simulink model "SIM_NonlinearPIwAW_2017b"  (R2017b)
settings: Solver=FixedStepAuto  StartTime=0.0  StopTime=9*0.25  FixedStep=h  RelTol=1e-3
values from neighbouring files (symbols this model uses):
  h = 1e-5    (= 1e-05)    [init.m]
  J = [0 -1; 1 0]    [generate_EKF.m]    (also in init.m)
  log_ts = 1e-5    (= 1e-05)    [init.m]
  lut_fr =     [friction.mat]
  omegam_ref = 157    [init.m]
  p = 2    [generate_EKF.m]
  P_init_dist = W_dist_noise    [init.m]
  pmsm_sew =     [config.mat]
  Psi_jac = [0.121, 0; 0, 0.0769]    [init.m]
  rsm_za =     [config.mat]
  SysConfig_SamplingTimeA = 0.00025    [config.mat]
  SysConfig_SamplingTimeB = 0.00025    [config.mat]
  u_DC = 556    [init.m]
  V_dist_noise = diag([2e0, 2e0])    [init.m]
  W_dist_noise = diag([1e-2, 1e-2, 1e4, 1e4])    [init.m]
  x_e_init_dist = zeros(4,1)    [init.m]
undefined symbols (not defined in the file or in its folder): DiscIntNeverNeededParam, f_pwm, k_i, k_p_tilde, uhat
libraries: simulink x4
(part 1 of 2)
settings Model: Creator=Julian Kullick  LastModifiedBy=andrea
settings DataIOCC: SaveFormat=StructureWithTime  SaveOutput=off  DSMLogging=off  SaveTime=off  SignalLoggingName=simData  LoggingFileName=./results/sim/NonlinearPIwAW.mat
settings SFSimCC: SimUseLocalCustomCode=on
settings RTWCC: RTWUseLocalCustomCode=on

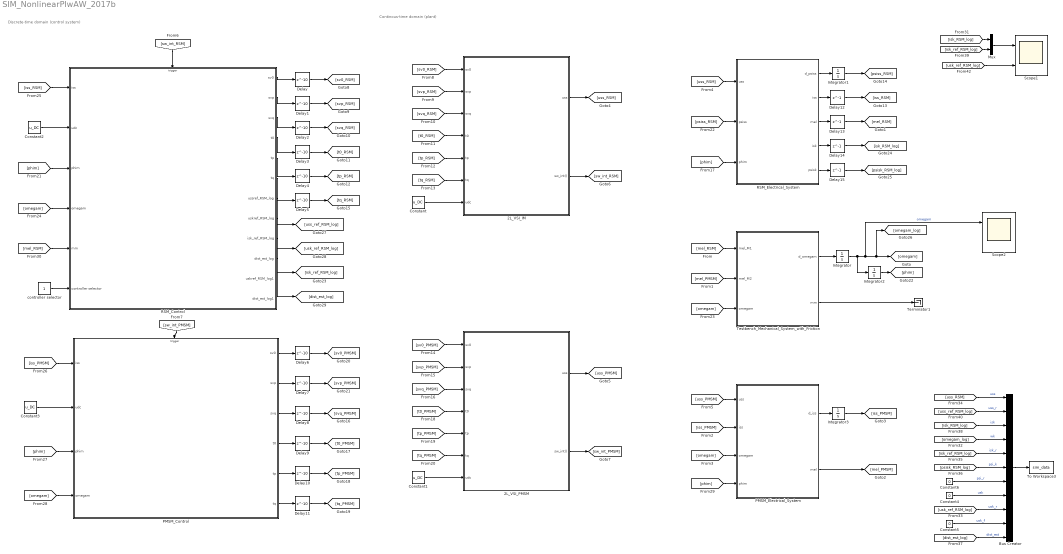
== system SIM_NonlinearPIwAW_2017b ==
  note: Continous-time domain (plant)
  note: Discrete-time domain (control system)
  2L_VSI_IM : Subsystem  mask{TS=SysConfig_SamplingTimeA, H=h}
      mask prompts: TS "PWM period (symmetric sampling)"; H "Model sampling time"
      mask DialogControl DescGroupVar Prompt: Description
      mask DialogControl DescTextVar Prompt: 2-level VSI output generator.
  2L_VSI_PMSM : Subsystem  mask{TS=SysConfig_SamplingTimeB, H=h}
      mask prompts: TS "PWM period (symmetric sampling)"; H "Model sampling time"
      mask DialogControl DescGroupVar Prompt: Description
      mask DialogControl DescTextVar Prompt: 2-level VSI output generator.
  Bus Creator : BusCreator  Inputs=11
  Constant{,1..3} (4 alike) : Constant  Value=u_DC
  Constant4 : Constant  Value=0
  Constant5 : Constant  Value=0
  Constant6 : Constant  Value=0
  Delay{,1..11} (12 alike) : Delay  DelayLength=10
  Delay{12..15} (4 alike) : Delay  DelayLength=1
  Integrator{,1..3} (4 alike) : Integrator
  Mux : Mux  Inputs=2
  PMSM_Control : Subsystem  TreatAsAtomicUnit=on
  PMSM_Electrical_System : MATLAB Function  TreatAsAtomicUnit=on  mask{RS=pmsm_sew.Rs, LS=pmsm_sew.Ls, PSIPM=pmsm_sew.PsiPM, NP=pmsm_sew.np}
      mask prompts: RS "Stator resistance (in Ohm)"; LS "Stator inductance (in H)"; PSIPM "Permanent magnet flux (in Wb)"; NP "Number of pole pairs"
  RSM_Control : Subsystem  TreatAsAtomicUnit=on
  RSM_Electrical_System : MATLAB Function  TreatAsAtomicUnit=on  mask{RS=rsm_za.Rs, NP=rsm_za.np, ISD=rsm_za.Is.d, ISQ=rsm_za.Is.q, PSISD=rsm_za.Psis.d, PSISQ=rsm_za.Psis.q}
      mask prompts: RS "Stator resistance (in Ohm)"; NP "Number of pole pairs"; ISD "d-Current for flux look-up (in A) [VEC]"; ISQ "q-Current for flux look-up (in A) [VEC]"; PSISD "d-Flux map (in Wb) [MAP]"; PSISQ "q-Flux map (in Wb) [MAP]|"
  Scope1 : Scope  NumInputPorts=2
  Scope2 : Scope  NumInputPorts=2
  Terminator1 : Terminator
  Testbench_Mechanical_System_with_Friction : MATLAB Function  TreatAsAtomicUnit=on  mask{THETAM_M1=rsm_za.Thetam, THETAM_M2=pmsm_sew.Thetam, MFR_LUT=lut_fr.m*0, WFR_LUT=lut_fr.omega}
      mask prompts: THETAM_M1 "Moment of inertia of machine 1 (in kg m^2)"; THETAM_M2 "Moment of inertia of machine 2 (in kg m^2)"; MFR_LUT "Friction torque [VEC] (in Nm)"; WFR_LUT "Speed vector for torque look-up [VEC] (in rad/s)"
  To Workspace3 : ToWorkspace  VariableName=sim_data  SaveFormat=Timeseries  SampleTime=log_ts
  controller selector : Constant
  wires:
  RSM_Electrical_System/1(d_psiss) -> Integrator1/1
  [phim] -> RSM_Electrical_System/3(phim)
  Integrator1/1 -> [psiss_RSM]
  RSM_Electrical_System/3(mel) -> Delay13/1
  [psiss_RSM] -> RSM_Electrical_System/2(psiss)
  Testbench_Mechanical_System_with_Friction/1(d_omegam) -> Integrator/1
  Integrator2/1 -> [phim]
  Testbench_Mechanical_System_with_Friction/2(mm) -> Terminator1/1
  PMSM_Electrical_System/2(mel) -> [mel_PMSM]
  Integrator3/1 -> [iss_PMSM]
  PMSM_Electrical_System/1(d_iss) -> Integrator3/1
  [iss_PMSM] -> PMSM_Electrical_System/2(iss)
  [omegam] -> PMSM_Electrical_System/3(omegam)
  2L_VSI_IM/1(uss) -> [uss_RSM]
  [uss_RSM] -> RSM_Electrical_System/1(uss)
  2L_VSI_PMSM/1(uss) -> [uss_PMSM]
  [uss_PMSM] -> PMSM_Electrical_System/1(uss)
  2L_VSI_IM/2(sw_int()) -> [sw_int_RSM]
  [sw_int_PMSM] -> PMSM_Control/Trigger
  2L_VSI_PMSM/2(sw_int()) -> [sw_int_PMSM]
  [sw_int_RSM] -> RSM_Control/Trigger
  RSM_Control/1(sv0) -> Delay/1
  RSM_Control/2(svp) -> Delay1/1
  RSM_Control/3(svq) -> Delay2/1
  RSM_Control/4(t0) -> Delay3/1
  RSM_Control/5(tp) -> Delay4/1
  RSM_Control/6(tq) -> Delay5/1
  [t0_RSM] -> 2L_VSI_IM/4(t0)
  [tq_RSM] -> 2L_VSI_IM/6(tq)
  [tp_RSM] -> 2L_VSI_IM/5(tp)
  [svq_RSM] -> 2L_VSI_IM/3(svq)
  [svp_RSM] -> 2L_VSI_IM/2(svp)
  [sv0_RSM] -> 2L_VSI_IM/1(sv0)
  Constant/1 -> 2L_VSI_IM/7(udc)
  PMSM_Control/1(sv0) -> Delay6/1
  PMSM_Control/2(svp) -> Delay7/1
  PMSM_Control/3(svq) -> Delay8/1
  PMSM_Control/4(t0) -> Delay9/1
  PMSM_Control/5(tp) -> Delay10/1
  PMSM_Control/6(tq) -> Delay11/1
  [sv0_PMSM] -> 2L_VSI_PMSM/1(sv0)
  [svp_PMSM] -> 2L_VSI_PMSM/2(svp)
  [svq_PMSM] -> 2L_VSI_PMSM/3(svq)
  [t0_PMSM] -> 2L_VSI_PMSM/4(t0)
  [tp_PMSM] -> 2L_VSI_PMSM/5(tp)
  [tq_PMSM] -> 2L_VSI_PMSM/6(tq)
  Constant1/1 -> 2L_VSI_PMSM/7(udc)
  [omegam] -> Testbench_Mechanical_System_with_Friction/3(omegam)
  Constant2/1 -> RSM_Control/2(udc)
  [omegam] -> RSM_Control/4(omegam)
  [iss_RSM] -> RSM_Control/1(iss)
  [iss_PMSM] -> PMSM_Control/1(iss)
  Constant3/1 -> PMSM_Control/2(udc)
  [phim] -> PMSM_Control/3(phim)
  [omegam] -> PMSM_Control/4(omegam)
  Integrator/1 -> Integrator2/1, Scope2/1, [omegam_log], [omegam]  "omegam"
  [mel_RSM] -> Testbench_Mechanical_System_with_Friction/1(mel_M1)
  [mel_PMSM] -> Testbench_Mechanical_System_with_Friction/2(mel_M2)
  [phim] -> PMSM_Electrical_System/4(phim)
  RSM_Electrical_System/2(iss) -> Delay12/1
  Delay/1 -> [sv0_RSM]
  Delay1/1 -> [svp_RSM]
  Delay2/1 -> [svq_RSM]
  Delay3/1 -> [t0_RSM]
  Delay4/1 -> [tp_RSM]
  Delay5/1 -> [tq_RSM]
  Delay6/1 -> [sv0_PMSM]
  Delay7/1 -> [svp_PMSM]
  Delay8/1 -> [svq_PMSM]
  Delay9/1 -> [t0_PMSM]
  Delay10/1 -> [tp_PMSM]
  Delay11/1 -> [tq_PMSM]
  Delay12/1 -> [iss_RSM]
  [phim] -> RSM_Control/3(phim)
  [mel_RSM] -> RSM_Control/5(mm)
  Delay13/1 -> [mel_RSM]
  controller selector/1 -> RSM_Control/6(controller selector)
  RSM_Electrical_System/4(isk) -> Delay14/1
  Delay14/1 -> [isk_RSM_log]
  RSM_Electrical_System/5(psisk) -> Delay15/1
  Delay15/1 -> [psisk_RSM_log]
  RSM_Control/7(ussref_RSM_log) -> [uss_ref_RSM_log]
  RSM_Control/8(uskref_RSM_log) -> [usk_ref_RSM_log]
  RSM_Control/9(isk_ref_RSM_log) -> [isk_ref_RSM_log]
  RSM_Control/10(dist_est_log) -> [dist_est_log]
  [isk_RSM_log] -> Mux/1
  [isk_ref_RSM_log] -> Mux/2
  [usk_ref_RSM_log] -> Scope1/2
  Mux/1 -> Scope1/1
  Bus Creator/1 -> To Workspace3/1
  [uss_RSM] -> Bus Creator/1  "uss"
  [uss_ref_RSM_log] -> Bus Creator/2  "uss_r"
  [isk_RSM_log] -> Bus Creator/3  "isk"
  [omegam_log] -> Bus Creator/4  "wk"
  [isk_ref_RSM_log] -> Bus Creator/5  "isk_r"
  [psisk_RSM_log] -> Bus Creator/6  "psi_k"
  Constant6/1 -> Bus Creator/7  "psi_r"
  Constant4/1 -> Bus Creator/8  "usk"
  [usk_ref_RSM_log] -> Bus Creator/9  "usk_r"
  Constant5/1 -> Bus Creator/10  "usk_f"
  [dist_est_log] -> Bus Creator/11  "dist_est"

== system SIM_NonlinearPIwAW_2017b/2L_VSI_IM ==
  sv0 : Inport
  svp : Inport  Port=2
  svq : Inport  Port=3
  t0 : Inport  Port=4
  tp : Inport  Port=5
  tq : Inport  Port=6
  udc : Inport  Port=7
  NL_VSI : Subsystem  mask{N=2, TPWM=TS, HSIM=H, INT_SHIFT=0}
      mask prompts: N "Number of levels"; TPWM "PWM period (symmetrical PWM)"; HSIM "Model sampling time"; INT_SHIFT "Interrupt shift (in percent of cycle time)"
      mask init:
      | INT_OFFSET = floor(TPWM/HSIM*INT_SHIFT*0.01);
      mask DialogControl DescTextVar Prompt: N-level VSI output signal generator.
  TC : Gain  Gain=2/3*[1 -0.5 -0.5; 0 sqrt(3)/2 -sqrt(3)/2]  Multiplication=Matrix(K*u)
  Terminator : Terminator
  uss : Outport
  sw_int() : Outport  Port=2
  wires:
  NL_VSI/3(sw_int()) -> sw_int()/1
  udc/1 -> NL_VSI/7(udc)
  NL_VSI/1(uabc0) -> TC/1
  sv0/1 -> NL_VSI/1(sv0)
  svp/1 -> NL_VSI/2(svp)
  svq/1 -> NL_VSI/3(svq)
  t0/1 -> NL_VSI/4(t0)
  tp/1 -> NL_VSI/5(tp)
  tq/1 -> NL_VSI/6(tq)
  TC/1 -> uss/1
  NL_VSI/2(ucm) -> Terminator/1

== system SIM_NonlinearPIwAW_2017b/2L_VSI_PMSM ==
  sv0 : Inport
  svp : Inport  Port=2
  svq : Inport  Port=3
  t0 : Inport  Port=4
  tp : Inport  Port=5
  tq : Inport  Port=6
  udc : Inport  Port=7
  NL_VSI : Subsystem  mask{N=2, TPWM=TS, HSIM=H, INT_SHIFT=0}
      mask prompts: N "Number of levels"; TPWM "PWM period (symmetrical PWM)"; HSIM "Model sampling time"; INT_SHIFT "Interrupt shift (in percent of cycle time)"
      mask init:
      | INT_OFFSET = floor(TPWM/HSIM*INT_SHIFT*0.01);
      mask DialogControl DescTextVar Prompt: N-level VSI output signal generator.
  TC : Gain  Gain=2/3*[1 -0.5 -0.5; 0 sqrt(3)/2 -sqrt(3)/2]  Multiplication=Matrix(K*u)
  Terminator : Terminator
  uss : Outport
  sw_int() : Outport  Port=2
  wires:
  NL_VSI/3(sw_int()) -> sw_int()/1
  udc/1 -> NL_VSI/7(udc)
  NL_VSI/1(uabc0) -> TC/1
  sv0/1 -> NL_VSI/1(sv0)
  svp/1 -> NL_VSI/2(svp)
  svq/1 -> NL_VSI/3(svq)
  t0/1 -> NL_VSI/4(t0)
  tp/1 -> NL_VSI/5(tp)
  tq/1 -> NL_VSI/6(tq)
  TC/1 -> uss/1
  NL_VSI/2(ucm) -> Terminator/1

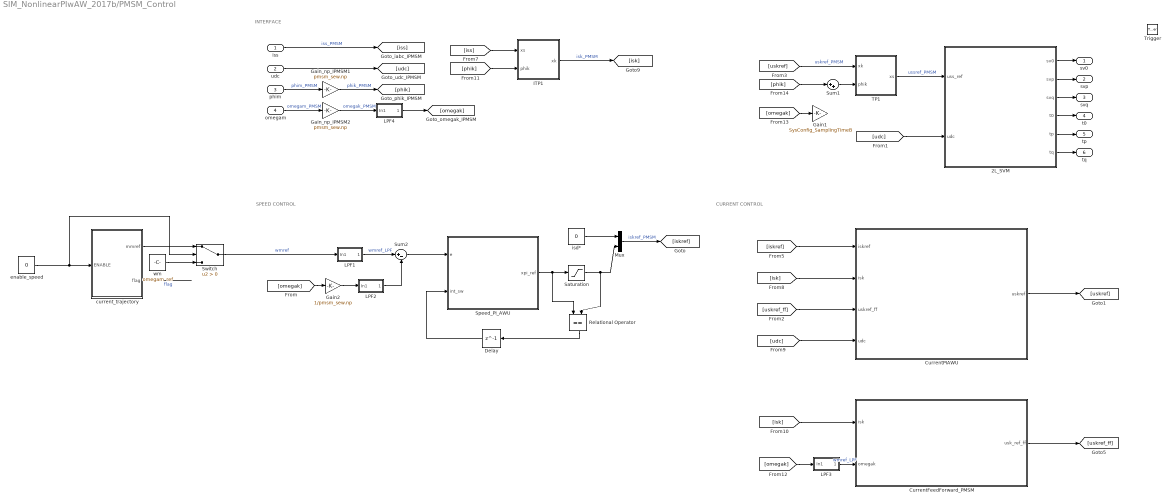
== system SIM_NonlinearPIwAW_2017b/PMSM_Control ==
  note: CURRENT CONTROL
  note: SPEED CONTROL
  note: INTERFACE
  iss : Inport
  udc : Inport  Port=2
  phim : Inport  Port=3
  omegam : Inport  Port=4
  Trigger : TriggerPort  TriggerType=function-call  VariantControl=Variant
  2L_SVM : Subsystem  mask{TS=SysConfig_SamplingTimeA}
      mask prompts: TS "PWM period (symmetric sampling)"
      mask DialogControl DescGroupVar Prompt: Description
      mask DialogControl DescTextVar Prompt: 2-level space vector modulator.
  CurrentFeedForward_PMSM : MATLAB Function  TreatAsAtomicUnit=on
  CurrentPIAWU : Subsystem  mask{VRD=pmsm_sew.VRis, TND=pmsm_sew.Tnis, VRQ=pmsm_sew.VRis, TNQ=pmsm_sew.Tnis}
      mask prompts: VRD "d-Current gain (constant part)"; TND "d-Current time constant (constant part)"; VRQ "q-Current gain (constant part)"; TNQ "q-Current time constant (constant part)"
      mask DialogControl DescGroupVar Prompt: Description
      mask DialogControl DescTextVar Prompt: Current control system with anti windup and online parameter adjustment.
  Delay : Delay  DelayLength=1
  Gain1 : Gain  Gain=SysConfig_SamplingTimeB
  Gain2 : Gain  Gain=1/pmsm_sew.np
  Gain_np_IPMSM1 : Gain  Gain=pmsm_sew.np
  Gain_np_IPMSM2 : Gain  Gain=pmsm_sew.np
  ITP1 : MATLAB Function  TreatAsAtomicUnit=on
  LPF1 : Subsystem  mask{TF=SysConfig_SamplingTimeB*100, TS=SysConfig_SamplingTimeB, SAT=inf}
      mask prompts: TF "Filter constant"; TS "Sampling time"; SAT "Saturation"
  LPF2 : Subsystem  mask{TF=SysConfig_SamplingTimeB*20, TS=SysConfig_SamplingTimeB, SAT=inf}
      mask prompts: TF "Filter constant"; TS "Sampling time"; SAT "Saturation"
  LPF3 : Subsystem  mask{TF=SysConfig_SamplingTimeB*10, TS=SysConfig_SamplingTimeB, SAT=350}
      mask prompts: TF "Filter constant"; TS "Sampling time"; SAT "Saturation"
  LPF4 : Subsystem  mask{TF=SysConfig_SamplingTimeB*32, TS=SysConfig_SamplingTimeB, SAT=inf}
      mask prompts: TF "Filter constant"; TS "Sampling time"; SAT "Saturation"
  Mux : Mux  Inputs=2
  Relational Operator : RelationalOperator  Operator===  OutDataTypeStr=boolean  RndMeth=Simplest
  Saturation : Saturate  UpperLimit=pmsm_sew.ishatN*1.2  LowerLimit=-pmsm_sew.ishatN*1.2
  Speed_PI_AWU : Subsystem  mask{VR=pmsm_sew.VRomegam*0.25, TN=pmsm_sew.Tnomegam*25}
      mask prompts: VR "Gain"; TN "Time constant (in s)"
  Sum1 : Sum  Inputs=|++
  Sum2 : Sum  Inputs=|+-
  Switch : Switch  Criteria=u2 > Threshold
  TP1 : MATLAB Function  TreatAsAtomicUnit=on
  current_trajectory : Subsystem
  enable_speed : Constant  Value=0
  isd* : Constant  Value=0
  wm : Constant  Value=omegam_ref
  sv0 : Outport
  svp : Outport  Port=2
  svq : Outport  Port=3
  t0 : Outport  Port=4
  tp : Outport  Port=5
  tq : Outport  Port=6
  wires:
  [omegak] -> LPF3/1(In1)
  Delay/1 -> Speed_PI_AWU/2(int_sw)
  [isk] -> CurrentPIAWU/2(isk)
  CurrentPIAWU/1(uskref) -> [uskref]
  Switch/1 -> LPF1/1(In1)  "wmref"
  [udc] -> CurrentPIAWU/4(udc)
  Speed_PI_AWU/1(xpi_ref) -> Relational Operator/1, Saturation/1
  [isk] -> CurrentFeedForward_PMSM/1(isk)
  Sum2/1 -> Speed_PI_AWU/1(e)
  Saturation/1 -> Relational Operator/2, Mux/2
  [uskref_ff] -> CurrentPIAWU/3(uskref_ff)
  [omegak] -> Gain2/1
  isd*/1 -> Mux/1
  CurrentFeedForward_PMSM/1(usk_ref_ff) -> [uskref_ff]
  Relational Operator/1 -> Delay/1
  2L_SVM/6(tq) -> tq/1
  2L_SVM/2(svp) -> svp/1
  2L_SVM/3(svq) -> svq/1
  2L_SVM/4(t0) -> t0/1
  2L_SVM/1(sv0) -> sv0/1
  2L_SVM/5(tp) -> tp/1
  Sum1/1 -> TP1/2(phik)
  ITP1/1(xk) -> [isk]  "isk_PMSM"
  [uskref] -> TP1/1(xk)  "uskref_PMSM"
  [phik] -> Sum1/1
  [phik] -> ITP1/2(phik)
  Gain_np_IPMSM1/1 -> [phik]  "phik_PMSM"
  [omegak] -> Gain1/1
  Gain_np_IPMSM2/1 -> LPF4/1(In1)  "omegak_PMSM"
  iss/1 -> [iss]  "iss_PMSM"
  [iss] -> ITP1/1(xs)
  udc/1 -> [udc]
  phim/1 -> Gain_np_IPMSM1/1  "phim_PMSM"
  omegam/1 -> Gain_np_IPMSM2/1  "omegam_PMSM"
  [udc] -> 2L_SVM/2(udc)
  TP1/1(xs) -> 2L_SVM/1(uss_ref)  "ussref_PMSM"
  Mux/1 -> [iskref]  "iskref_PMSM"
  Gain2/1 -> LPF2/1(In1)
  [iskref] -> CurrentPIAWU/1(iskref)
  LPF1/1(Out1) -> Sum2/1  "wmref_LPF"
  LPF2/1(Out1) -> Sum2/2
  current_trajectory/2(flag) -> ?  "flag"
  wm/1 -> Switch/3
  current_trajectory/1(mmref) -> Switch/1
  enable_speed/1 -> Switch/2, current_trajectory/1(ENABLE)
  LPF3/1(Out1) -> CurrentFeedForward_PMSM/2(omegak)  "wmref_LPF"
  LPF4/1(Out1) -> [omegak]

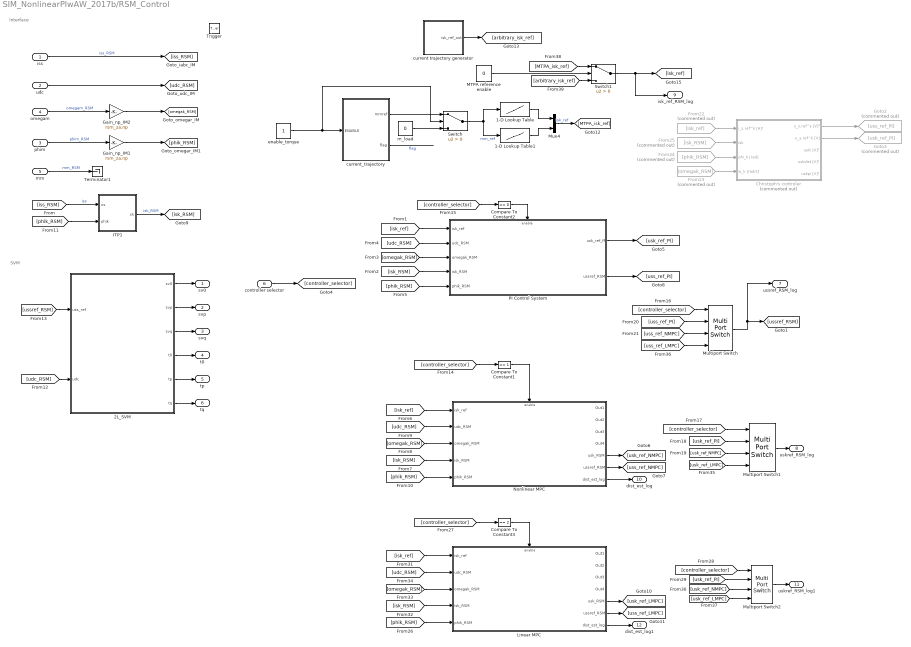
== system SIM_NonlinearPIwAW_2017b/RSM_Control ==
  note: SVM
  note: Interface
  iss : Inport
  udc : Inport  Port=2
  phim : Inport  Port=3
  omegam : Inport  Port=4
  mm : Inport  Port=5
  controller selector : Inport  Port=6
  Trigger : TriggerPort  TriggerType=function-call  VariantControl=Variant
  1-D Lookup Table : Lookup_n-D  NumberOfTableDimensions=1  BreakpointsForDimension1=rsm_za.MTPA.mm  Table=rsm_za.MTPA.d  RemoveProtectionInput=on  InternalRulePriority=Speed  RndMeth=Simplest  InputSameDT=on
  1-D Lookup Table1 : Lookup_n-D  NumberOfTableDimensions=1  BreakpointsForDimension1=rsm_za.MTPA.mm  Table=rsm_za.MTPA.q  RemoveProtectionInput=on  InternalRulePriority=Speed  RndMeth=Simplest  InputSameDT=on
  2L_SVM : Subsystem  mask{TS=SysConfig_SamplingTimeA}
      mask prompts: TS "PWM period (symmetric sampling)"
      mask DialogControl DescGroupVar Prompt: Description
      mask DialogControl DescTextVar Prompt: 2-level space vector modulator.
  Christoph's controler : Subsystem  Commented=on
  Compare To Constant1 : simulink/Logic and Bit Operations/Compare To Constant  relop===  const=1  OutDataTypeStr=boolean
  Compare To Constant2 : simulink/Logic and Bit Operations/Compare To Constant  relop===  const=0  OutDataTypeStr=boolean
  Compare To Constant3 : simulink/Logic and Bit Operations/Compare To Constant  relop===  const=2  OutDataTypeStr=boolean
  From22 : From  Commented=on  GotoTag=isk_ref
  From23 : From  Commented=on  GotoTag=omegak_RSM
  From24 : From  Commented=on  GotoTag=phik_RSM
  From25 : From  Commented=on  GotoTag=isk_RSM
  Gain_np_IM1 : Gain  Gain=rsm_za.np
  Gain_np_IM2 : Gain  Gain=rsm_za.np
  Goto2 : Goto  Commented=on  GotoTag=uss_ref_PI
  Goto3 : Goto  Commented=on  GotoTag=usk_ref_PI
  ITP1 : MATLAB Function  TreatAsAtomicUnit=on
  Linear MPC : Subsystem
  MTPA reference enable : Constant  Value=0
  Multiport Switch : MultiPortSwitch  DataPortOrder=Zero-based contiguous  zeroidx=on
  Multiport Switch1 : MultiPortSwitch  DataPortOrder=Zero-based contiguous  zeroidx=on
  Multiport Switch2 : MultiPortSwitch  DataPortOrder=Zero-based contiguous  zeroidx=on
  Mux4 : Mux  Inputs=2
  Nonlinear MPC : Subsystem
  PI Control System : Subsystem
  Switch : Switch  Criteria=u2 > Threshold
  Switch1 : Switch  Criteria=u2 > Threshold
  Terminator1 : Terminator
  current trajectory generator : Subsystem
  current_trajectory : Subsystem
  enable_torque : Constant
  m_load : Constant  Value=0
  sv0 : Outport
  svp : Outport  Port=2
  svq : Outport  Port=3
  t0 : Outport  Port=4
  tp : Outport  Port=5
  tq : Outport  Port=6
  ussref_RSM_log : Outport  Port=7
  uskref_RSM_log : Outport  Port=8
  isk_ref_RSM_log : Outport  Port=9
  dist_est_log : Outport  Port=10
  uskref_RSM_log1 : Outport  Port=11
  dist_est_log1 : Outport  Port=12
  wires:
  2L_SVM/1(sv0) -> sv0/1
  2L_SVM/2(svp) -> svp/1
  2L_SVM/3(svq) -> svq/1
  2L_SVM/4(t0) -> t0/1
  2L_SVM/5(tp) -> tp/1
  2L_SVM/6(tq) -> tq/1
  [udc_RSM] -> 2L_SVM/2(udc)
  udc/1 -> [udc_RSM]
  Gain_np_IM2/1 -> [omegak_RSM]
  iss/1 -> [iss_RSM]  "iss_RSM"
  omegam/1 -> Gain_np_IM2/1  "omegam_RSM"
  [ussref_RSM] -> 2L_SVM/1(uss_ref)
  Gain_np_IM1/1 -> [phik_RSM]
  phim/1 -> Gain_np_IM1/1  "phim_RSM"
  mm/1 -> Terminator1/1  "mm_RSM"
  current_trajectory/1(mmref) -> Switch/1
  current_trajectory/2(flag) -> ?  "flag"
  m_load/1 -> Switch/3
  1-D Lookup Table/1 -> Mux4/1
  enable_torque/1 -> Switch/2, current_trajectory/1(ENABLE)
  Switch/1 -> 1-D Lookup Table1/1, 1-D Lookup Table/1  "mm_ref"
  1-D Lookup Table1/1 -> Mux4/2
  [iss_RSM] -> ITP1/1(xs)  "iss"
  ITP1/1(xk) -> [isk_RSM]  "isk_RSM"
  [phik_RSM] -> ITP1/2(phik)
  Compare To Constant2/1 -> PI Control System/Enable
  Compare To Constant1/1 -> Nonlinear MPC/Enable
  [isk_ref] -> PI Control System/1(isk_ref)
  [isk_RSM] -> PI Control System/4(isk_RSM)
  [omegak_RSM] -> PI Control System/3(omegak_RSM)
  [udc_RSM] -> PI Control System/2(udc_RSM)
  [phik_RSM] -> PI Control System/5(phik_RSM)
  PI Control System/1(usk_ref_ff) -> [usk_ref_PI]
  [isk_RSM] -> Nonlinear MPC/4(isk_RSM)
  [phik_RSM] -> Nonlinear MPC/5(phik_RSM)
  [isk_ref] -> Nonlinear MPC/1(isk_ref)
  [udc_RSM] -> Nonlinear MPC/2(udc_RSM)
  [omegak_RSM] -> Nonlinear MPC/3(omegak_RSM)
  Multiport Switch/1 -> ussref_RSM_log/1, [ussref_RSM]
  [controller_selector] -> Compare To Constant1/1
  [controller_selector] -> Compare To Constant2/1
  controller selector/1 -> [controller_selector]
  [controller_selector] -> Multiport Switch/1
  [controller_selector] -> Multiport Switch1/1
  [usk_ref_PI] -> Multiport Switch1/2
  Nonlinear MPC/5(usk_RSM) -> [usk_ref_NMPC]
  [usk_ref_NMPC] -> Multiport Switch1/3
  Nonlinear MPC/6(ussref_RSM) -> [uss_ref_NMPC]
  PI Control System/2(ussref_RSM) -> [uss_ref_PI]
  [uss_ref_PI] -> Multiport Switch/2
  [uss_ref_NMPC] -> Multiport Switch/3
  Multiport Switch1/1 -> uskref_RSM_log/1
  Nonlinear MPC/7(dist_est_log) -> dist_est_log/1
  From22/1 -> Christoph's controler/1(i_s,ref^k [A]²)
  From23/1 -> Christoph's controler/4(w_k [rad/s])
  From24/1 -> Christoph's controler/3(phi_k [rad])
  From25/1 -> Christoph's controler/2(isk)
  Christoph's controler/1(u_s,ref^s [V]²) -> Goto2/1
  Christoph's controler/2(u_s,ref^k [V]) -> Goto3/1
  [controller_selector] -> Compare To Constant3/1
  Compare To Constant3/1 -> Linear MPC/Enable
  [phik_RSM] -> Linear MPC/5(phik_RSM)
  Linear MPC/5(usk_RSM) -> [usk_ref_LMPC]
  [isk_ref] -> Linear MPC/1(isk_ref)
  [usk_ref_NMPC] -> Multiport Switch2/3
  Linear MPC/6(ussref_RSM) -> [uss_ref_LMPC]
  Multiport Switch2/1 -> uskref_RSM_log1/1
  [usk_ref_PI] -> Multiport Switch2/2
  Linear MPC/7(dist_est_log) -> dist_est_log1/1
  [omegak_RSM] -> Linear MPC/3(omegak_RSM)
  [controller_selector] -> Multiport Switch2/1
  [udc_RSM] -> Linear MPC/2(udc_RSM)
  [isk_RSM] -> Linear MPC/4(isk_RSM)
  [usk_ref_LMPC] -> Multiport Switch1/4
  [uss_ref_LMPC] -> Multiport Switch/4
  [usk_ref_LMPC] -> Multiport Switch2/4
  Switch1/1 -> isk_ref_RSM_log/1, [isk_ref]
  Mux4/1 -> [MTPA_isk_ref]  "isk_ref"
  [MTPA_isk_ref] -> Switch1/1
  MTPA reference enable/1 -> Switch1/2
  current trajectory generator/1(isk_ref_out) -> [arbitrary_isk_ref]
  [arbitrary_isk_ref] -> Switch1/3

== system SIM_NonlinearPIwAW_2017b/2L_VSI_IM/NL_VSI ==
  sv0 : Inport
  svp : Inport  Port=2
  svq : Inport  Port=3
  t0 : Inport  Port=4
  tp : Inport  Port=5
  tq : Inport  Port=6
  udc : Inport  Port=7
  NL_VSI : MATLAB Function  TreatAsAtomicUnit=on
  uabc0 : Outport
  ucm : Outport  Port=2
  sw_int() : Outport  Port=3
  wires:
  NL_VSI/2(ucm) -> ucm/1
  tq/1 -> NL_VSI/6(tq)
  NL_VSI/3(sw_int()) -> sw_int()/1
  t0/1 -> NL_VSI/4(t0)
  svq/1 -> NL_VSI/3(svq)
  sv0/1 -> NL_VSI/1(sv0)
  NL_VSI/1(uabc0) -> uabc0/1
  tp/1 -> NL_VSI/5(tp)
  udc/1 -> NL_VSI/7(udc)
  svp/1 -> NL_VSI/2(svp)

== system SIM_NonlinearPIwAW_2017b/2L_VSI_PMSM/NL_VSI ==
  sv0 : Inport
  svp : Inport  Port=2
  svq : Inport  Port=3
  t0 : Inport  Port=4
  tp : Inport  Port=5
  tq : Inport  Port=6
  udc : Inport  Port=7
  NL_VSI : MATLAB Function  TreatAsAtomicUnit=on
  uabc0 : Outport
  ucm : Outport  Port=2
  sw_int() : Outport  Port=3
  wires:
  NL_VSI/2(ucm) -> ucm/1
  tq/1 -> NL_VSI/6(tq)
  NL_VSI/3(sw_int()) -> sw_int()/1
  t0/1 -> NL_VSI/4(t0)
  svq/1 -> NL_VSI/3(svq)
  sv0/1 -> NL_VSI/1(sv0)
  NL_VSI/1(uabc0) -> uabc0/1
  tp/1 -> NL_VSI/5(tp)
  udc/1 -> NL_VSI/7(udc)
  svp/1 -> NL_VSI/2(svp)

== system SIM_NonlinearPIwAW_2017b/PMSM_Control/2L_SVM ==
  uss_ref : Inport
  udc : Inport  Port=2
  2L_SVM : MATLAB Function  TreatAsAtomicUnit=on  mask{N=2, TPWM=TS}
      mask prompts: N "Number of levels"; TPWM "PWM period (symmetrical PWM)"
  sv0 : Outport
  svp : Outport  Port=2
  svq : Outport  Port=3
  t0 : Outport  Port=4
  tp : Outport  Port=5
  tq : Outport  Port=6
  wires:
  uss_ref/1 -> 2L_SVM/1(uab_ref)
  udc/1 -> 2L_SVM/2(udc)
  2L_SVM/1(sv0) -> sv0/1
  2L_SVM/2(svp) -> svp/1
  2L_SVM/3(svq) -> svq/1
  2L_SVM/4(t0) -> t0/1
  2L_SVM/5(tp) -> tp/1
  2L_SVM/6(tq) -> tq/1

== system SIM_NonlinearPIwAW_2017b/PMSM_Control/CurrentPIAWU ==
  iskref : Inport
  isk : Inport  Port=2
  uskref_ff : Inport  Port=3
  udc : Inport  Port=4
  Demux : Demux  Outputs=2
  Mux1 : Mux  Inputs=2
  Sum : Sum  Inputs=++|
  Sum1 : Sum  Inputs=+|-
  Voltage_Saturation : MATLAB Function  TreatAsAtomicUnit=on
  d_Current_PI_AWU_VRA : Subsystem  mask{VR=VRD, TN=TND}
      mask prompts: VR "Constant part of Proportional Gain K_p"; TN "Time Constant T_I"
      mask DialogControl DescGroupVar Prompt: Description
      mask DialogControl DescTextVar Prompt: PI-current controller with anti windup and parameter adaption.
  q_Current_PI_AWU_VRA : Subsystem  mask{VR=VRQ, TN=TNQ}
      mask prompts: VR "Constant part of Proportional Gain K_p"; TN "Time Constant T_I"
      mask DialogControl DescGroupVar Prompt: Description
      mask DialogControl DescTextVar Prompt: PI-current controller with anti windup and parameter adaption.
  uskref : Outport
  wires:
  Sum1/1 -> Demux/1
  isk/1 -> Sum1/2
  iskref/1 -> Sum1/1
  [int_sw] -> d_Current_PI_AWU_VRA/2(int_sw)
  Demux/1 -> d_Current_PI_AWU_VRA/1(e)
  Sum/1 -> Voltage_Saturation/1(usk)
  q_Current_PI_AWU_VRA/1(xpi_ref) -> Mux1/2
  Voltage_Saturation/2(int_sw) -> [int_sw]
  uskref_ff/1 -> Sum/1
  Mux1/1 -> Sum/2
  Voltage_Saturation/1(usk_sat) -> uskref/1
  [int_sw] -> q_Current_PI_AWU_VRA/2(int_sw)
  d_Current_PI_AWU_VRA/1(xpi_ref) -> Mux1/1
  Demux/2 -> q_Current_PI_AWU_VRA/1(e)
  udc/1 -> Voltage_Saturation/2(udc)

== system SIM_NonlinearPIwAW_2017b/PMSM_Control/LPF1 ==
  In1 : Inport
  Delay : Delay  DelayLength=1
  Delay1 : Delay  DelayLength=1
  Gain : Gain  Gain=1-2*TF/TS
  Gain1 : Gain  Gain=1/(1+2*TF/TS)
  Saturation : Saturate  UpperLimit=SAT  LowerLimit=-SAT
  Sum : Sum  Inputs=++-
  Out1 : Outport
  wires:
  Saturation/1 -> Out1/1
  In1/1 -> Delay1/1, Sum/2
  Sum/1 -> Gain1/1
  Delay1/1 -> Sum/1
  Gain/1 -> Sum/3
  Gain1/1 -> Delay/1
  Delay/1 -> Gain/1, Saturation/1

== system SIM_NonlinearPIwAW_2017b/PMSM_Control/LPF2 ==
  In1 : Inport
  Delay : Delay  DelayLength=1
  Delay1 : Delay  DelayLength=1
  Gain : Gain  Gain=1-2*TF/TS
  Gain1 : Gain  Gain=1/(1+2*TF/TS)
  Saturation : Saturate  UpperLimit=SAT  LowerLimit=-SAT
  Sum : Sum  Inputs=++-
  Out1 : Outport
  wires:
  Delay/1 -> Saturation/1, Gain/1
  Gain1/1 -> Delay/1
  Gain/1 -> Sum/3
  Delay1/1 -> Sum/1
  Sum/1 -> Gain1/1
  In1/1 -> Sum/2, Delay1/1
  Saturation/1 -> Out1/1

== system SIM_NonlinearPIwAW_2017b/PMSM_Control/LPF3 ==
  In1 : Inport
  Delay : Delay  DelayLength=1
  Delay1 : Delay  DelayLength=1
  Gain : Gain  Gain=1-2*TF/TS
  Gain1 : Gain  Gain=1/(1+2*TF/TS)
  Saturation : Saturate  UpperLimit=SAT  LowerLimit=-SAT
  Sum : Sum  Inputs=++-
  Out1 : Outport
  wires:
  Delay/1 -> Saturation/1, Gain/1
  Gain1/1 -> Delay/1
  Gain/1 -> Sum/3
  Delay1/1 -> Sum/1
  Sum/1 -> Gain1/1
  In1/1 -> Sum/2, Delay1/1
  Saturation/1 -> Out1/1

== system SIM_NonlinearPIwAW_2017b/PMSM_Control/LPF4 ==
  In1 : Inport
  Delay : Delay  DelayLength=1
  Delay1 : Delay  DelayLength=1
  Gain : Gain  Gain=1-2*TF/TS
  Gain1 : Gain  Gain=1/(1+2*TF/TS)
  Saturation : Saturate  UpperLimit=SAT  LowerLimit=-SAT
  Sum : Sum  Inputs=++-
  Out1 : Outport
  wires:
  Saturation/1 -> Out1/1
  In1/1 -> Delay1/1, Sum/2
  Sum/1 -> Gain1/1
  Delay1/1 -> Sum/1
  Gain/1 -> Sum/3
  Gain1/1 -> Delay/1
  Delay/1 -> Gain/1, Saturation/1

== system SIM_NonlinearPIwAW_2017b/PMSM_Control/Speed_PI_AWU ==
  e : Inport
  int_sw : Inport  Port=2
  1/Tn : Gain  Gain=1/TN
  Constant : Constant  Value=0
  Discrete-Time Integrator : DiscreteIntegrator  SampleTime=-1  ICPrevOutput=DiscIntNeverNeededParam  ICPrevScaledInput=DiscIntNeverNeededParam
  Sum : Sum  Inputs=|++
  Switch : Switch  Criteria=u2 > Threshold
  VR : Gain  Gain=VR
  xpi_ref : Outport  OutputWhenDisabled=reset  InitialOutput=[0]
  wires:
  1/Tn/1 -> Switch/1
  Switch/1 -> Discrete-Time Integrator/1
  e/1 -> VR/1
  int_sw/1 -> Switch/2
  Sum/1 -> xpi_ref/1
  Constant/1 -> Switch/3
  Discrete-Time Integrator/1 -> Sum/2
  VR/1 -> 1/Tn/1, Sum/1

== system SIM_NonlinearPIwAW_2017b/PMSM_Control/current_trajectory ==
  ENABLE : Inport
  Product : Product
  REF_GEN : MATLAB Function  TreatAsAtomicUnit=on
  duration : Constant  Value=2
  wmmax : Constant  Value=157
  xvecp : Constant  Value=[0 0.5 0.25 1 0 -1 -0.25 -0.5 0]
  mmref : Outport
  flag : Outport  Port=2
  wires:
  ENABLE/1 -> REF_GEN/1(ENABLE_FLAG)
  REF_GEN/2(active_flag) -> flag/1
  REF_GEN/1(mmref) -> mmref/1
  xvecp/1 -> Product/1
  Product/1 -> REF_GEN/2(xvec)
  wmmax/1 -> Product/2
  duration/1 -> REF_GEN/3(duration)

== system SIM_NonlinearPIwAW_2017b/RSM_Control/2L_SVM ==
  uss_ref : Inport
  udc : Inport  Port=2
  2L_SVM : MATLAB Function  TreatAsAtomicUnit=on  mask{N=2, TPWM=TS}
      mask prompts: N "Number of levels"; TPWM "PWM period (symmetrical PWM)"
  sv0 : Outport
  svp : Outport  Port=2
  svq : Outport  Port=3
  t0 : Outport  Port=4
  tp : Outport  Port=5
  tq : Outport  Port=6
  wires:
  uss_ref/1 -> 2L_SVM/1(uab_ref)
  udc/1 -> 2L_SVM/2(udc)
  2L_SVM/1(sv0) -> sv0/1
  2L_SVM/2(svp) -> svp/1
  2L_SVM/3(svq) -> svq/1
  2L_SVM/4(t0) -> t0/1
  2L_SVM/5(tp) -> tp/1
  2L_SVM/6(tq) -> tq/1

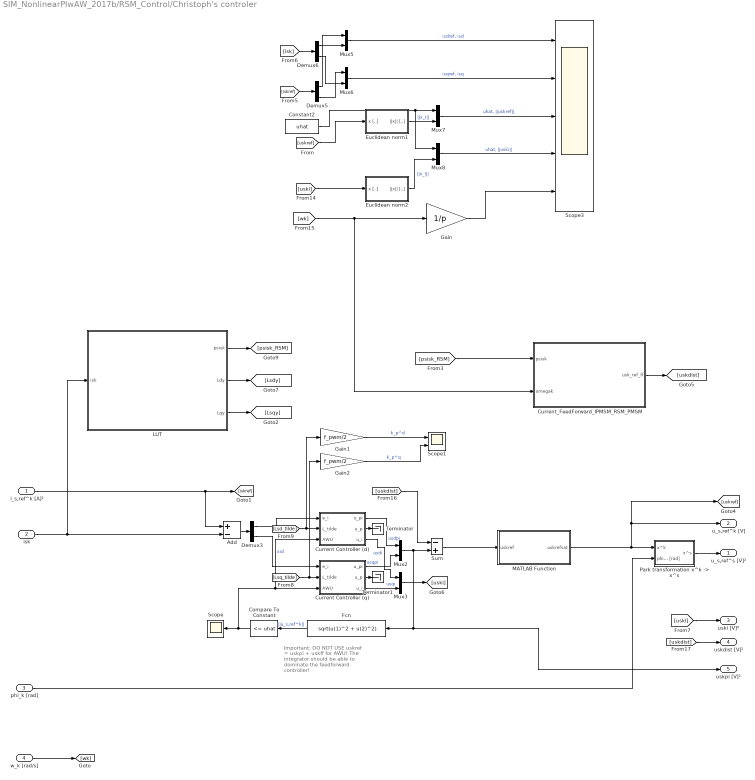
== system SIM_NonlinearPIwAW_2017b/RSM_Control/Christoph's controler ==
  note: Important: DO NOT USE uskref = uskpi + uskff for AWU!
      | The integrator should be able to dominate the feedforward controller!
  i_s,ref^k [A]² : Inport
  isk : Inport  Port=2
  phi_k [rad] : Inport  Port=3
  w_k [rad/s] : Inport  Port=4
  Add : Sum  Inputs=+-
  Compare To Constant : simulink/Logic and Bit Operations/Compare To Constant  relop=<=  const=uhat  OutDataTypeStr=boolean
  Constant2 : Constant  Value=uhat
  Current Controller (d) : Subsystem  mask{P_GAIN=k_p_tilde, I_GAIN=k_i, INT_INIT=0}
      mask prompts: P_GAIN "Proportional gain k_p"; I_GAIN "Integral gain k_I"; INT_INIT "Initial condition"
      mask DialogControl DescGroupVar Prompt: Adaptive PI Controller
      mask DialogControl DescTextVar Prompt: A simple PI-Controller with Anti Windup
  Current Controller (q) : Subsystem  mask{P_GAIN=k_p_tilde, I_GAIN=k_i, INT_INIT=0}
      mask prompts: P_GAIN "Proportional gain k_p"; I_GAIN "Integral gain k_I"; INT_INIT "Initial condition"
      mask DialogControl DescGroupVar Prompt: Adaptive PI Controller
      mask DialogControl DescTextVar Prompt: A simple PI-Controller with Anti Windup
  Current_FeedForward_IPMSM_RSM_PMSM : MATLAB Function  TreatAsAtomicUnit=on
  Demux3 : Demux  Outputs=2
  Demux5 : Demux  Outputs=2
  Demux6 : Demux  Outputs=2
  Euclidean norm1 : Subsystem
  Euclidean norm2 : Subsystem
  Fcn : Fcn  Expr=sqrt(u(1)^2 + u(2)^2)
  Gain : Gain  Gain=1/p
  Gain1 : Gain  Gain=f_pwm/2
  Gain2 : Gain  Gain=f_pwm/2
  LUT : Subsystem
  MATLAB Function : MATLAB Function  TreatAsAtomicUnit=on
  Mux{2..3,5..8} (6 alike) : Mux  Inputs=2
  "Park transformation x^k -> x^s" : Subsystem
  Scope : Scope
  Scope1 : Scope  NumInputPorts=2
  Scope3 : Scope  NumInputPorts=5
  Sum : Sum  Inputs=-+
  Terminator : Terminator
  Terminator1 : Terminator
  u_s,ref^s [V]² : Outport
  u_s,ref^k [V] : Outport  Port=2
  uski [V]² : Outport  Port=3
  uskdist [V]² : Outport  Port=4
  uskpi [V]² : Outport  Port=5
  wires:
  phi_k [rad]/1 -> "Park transformation x^k -> x^s"/2(phi_k [rad])
  "Park transformation x^k -> x^s"/1(x^s) -> u_s,ref^s [V]²/1
  Sum/1 -> MATLAB Function/1(uskref)
  [Lsd_tilde] -> Gain1/1, Current Controller (d)/2(L_tilde)
  [Lsq_tilde] -> Gain2/1, Current Controller (q)/2(L_tilde)
  Current Controller (d)/1(u_pi) -> Mux2/1  "usdpi"
  Current Controller (q)/1(u_pi) -> Mux2/2  "usqpi"
  Demux3/1 -> Current Controller (d)/1(e_i)
  Add/1 -> Demux3/1
  Demux3/2 -> Current Controller (q)/1(e_i)
  Fcn/1 -> Compare To Constant/1  "||u_s,ref^k||"
  i_s,ref^k [A]²/1 -> Add/1, [iskref]
  w_k [rad/s]/1 -> [wk]
  [uskref] -> Euclidean norm1/1(x [..])
  [isk] -> Demux6/1
  Euclidean norm1/1(||x|| [..]) -> Mux7/2  "||x_I||"
  Mux5/1 -> Scope3/1  "isdref, isd"
  [uski] -> Euclidean norm2/1(x [..])
  Mux8/1 -> Scope3/4  "uhat, ||uski||"
  Demux5/2 -> Mux6/1
  Euclidean norm2/1(||x|| [..]) -> Mux8/2  "||x_I||"
  [iskref] -> Demux5/1
  Gain/1 -> Scope3/5
  Demux6/2 -> Mux6/2
  Demux6/1 -> Mux5/2
  Mux7/1 -> Scope3/3  "uhat, ||uskref||"
  Demux5/1 -> Mux5/1
  Constant2/1 -> Mux8/1, Mux7/1
  Mux6/1 -> Scope3/2  "isqref, isq"
  Current Controller (q)/3(u_i) -> Mux3/2  "usqi"
  Compare To Constant/1 -> Scope/1, Current Controller (d)/3(AWU), Current Controller (q)/3(AWU)  "xid"
  Mux3/1 -> [uski]
  Current Controller (d)/3(u_i) -> Mux3/1  "usdi"
  Mux2/1 -> uskpi [V]²/1, Fcn/1, Sum/2
  Current Controller (d)/2(u_p) -> Terminator/1
  Current Controller (q)/2(u_p) -> Terminator1/1
  MATLAB Function/1(uskrefsat) -> u_s,ref^k [V]/1, [uskref], "Park transformation x^k -> x^s"/1(x^k)
  [uski] -> uski [V]²/1
  [uskdist] -> uskdist [V]²/1
  Gain1/1 -> Scope1/1  "k_p^d"
  Gain2/1 -> Scope1/2  "k_p^q"
  [psisk_RSM] -> Current_FeedForward_IPMSM_RSM_PMSM/1(psisk)
  Current_FeedForward_IPMSM_RSM_PMSM/1(usk_ref_ff) -> [uskdist]
  [wk] -> Current_FeedForward_IPMSM_RSM_PMSM/2(omegak), Gain/1
  LUT/3(Lqy) -> [Lsqy]
  LUT/1(psisk) -> [psisk_RSM]
  LUT/2(Ldy) -> [Lsdy]
  isk/1 -> LUT/1(isk), Add/2
  [uskdist] -> Sum/1

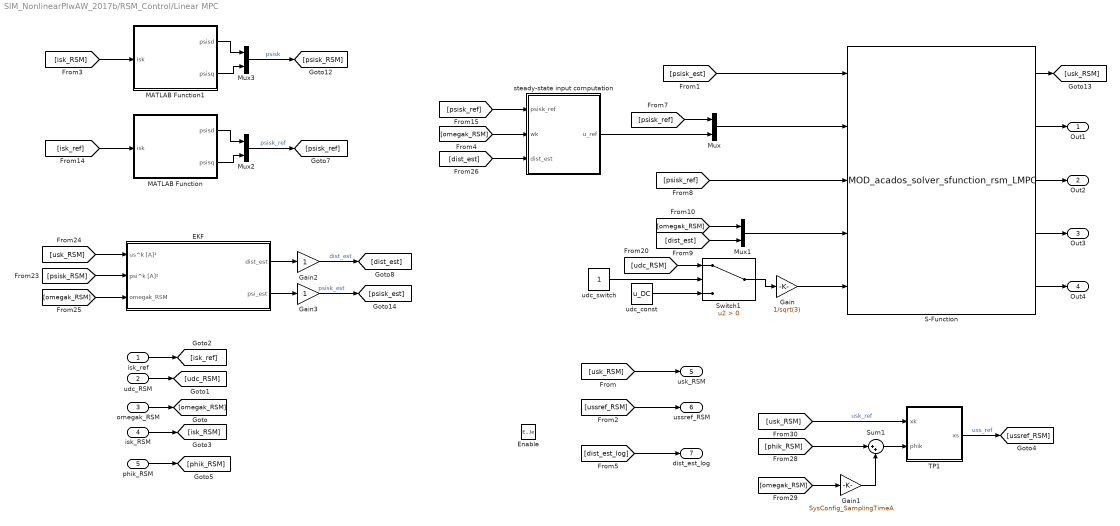
== system SIM_NonlinearPIwAW_2017b/RSM_Control/Linear MPC ==
  isk_ref : Inport
  udc_RSM : Inport  Port=2
  omegak_RSM : Inport  Port=3
  isk_RSM : Inport  Port=4
  phik_RSM : Inport  Port=5
  Enable : EnablePort
  "EKF " : Subsystem
  Gain : Gain  Gain=1/sqrt(3)
  Gain1 : Gain  Gain=SysConfig_SamplingTimeA
  Gain2 : Gain
  Gain3 : Gain
  MATLAB Function : MATLAB Function  TreatAsAtomicUnit=on
  MATLAB Function1 : MATLAB Function  TreatAsAtomicUnit=on
  Mux{,1..3} (4 alike) : Mux  Inputs=2
  S-Function : S-Function  FunctionName=MOD_acados_solver_sfunction_rsm_LMPC  SFunctionDeploymentMode=off  EnableBusSupport=off
  Sum1 : Sum  Inputs=|++
  Switch1 : Switch  Criteria=u2 > Threshold
  TP1 : MATLAB Function  TreatAsAtomicUnit=on
  steady-state input computation : Subsystem
  udc_const : Constant  Value=u_DC
  udc_switch : Constant
  Out1 : Outport
  Out2 : Outport  Port=2
  Out3 : Outport  Port=3
  Out4 : Outport  Port=4
  usk_RSM : Outport  Port=5
  ussref_RSM : Outport  Port=6
  dist_est_log : Outport  Port=7
  wires:
  S-Function/3 -> Out2/1
  S-Function/1 -> [usk_RSM]
  [psisk_ref] -> steady-state input computation/1(psisk_ref)
  [dist_est] -> steady-state input computation/3(dist_est)
  Gain2/1 -> [dist_est]  "dist_est"
  S-Function/2 -> Out1/1
  [udc_RSM] -> Switch1/1
  [isk_ref] -> MATLAB Function/1(isk)
  [psisk_RSM] -> "EKF "/2(psi^k [A]²)
  [psisk_est] -> S-Function/1
  Mux/1 -> S-Function/2
  Gain/1 -> S-Function/5
  Switch1/1 -> Gain/1
  [dist_est] -> Mux1/2
  [isk_RSM] -> MATLAB Function1/1(isk)
  MATLAB Function1/1(psisd) -> Mux3/1
  [psisk_ref] -> Mux/1
  MATLAB Function1/2(psisq) -> Mux3/2
  S-Function/5 -> Out4/1
  [omegak_RSM] -> "EKF "/3(omegak_RSM)
  [omegak_RSM] -> Mux1/1
  Mux3/1 -> [psisk_RSM]  "psisk"
  udc_switch/1 -> Switch1/2
  MATLAB Function/1(psisd) -> Mux2/1
  [usk_RSM] -> "EKF "/1(us^k [A]²)
  S-Function/4 -> Out3/1
  udc_const/1 -> Switch1/3
  steady-state input computation/1(u_ref) -> Mux/2
  Mux1/1 -> S-Function/4
  Gain3/1 -> [psisk_est]  "psisk_est"
  Mux2/1 -> [psisk_ref]  "psisk_ref"
  "EKF "/1(dist_est) -> Gain2/1
  "EKF "/2(psi_est) -> Gain3/1
  [omegak_RSM] -> steady-state input computation/2(wk)
  MATLAB Function/2(psisq) -> Mux2/2
  [psisk_ref] -> S-Function/3
  isk_ref/1 -> [isk_ref]
  isk_RSM/1 -> [isk_RSM]
  omegak_RSM/1 -> [omegak_RSM]
  phik_RSM/1 -> [phik_RSM]
  udc_RSM/1 -> [udc_RSM]
  [usk_RSM] -> usk_RSM/1
  Gain1/1 -> Sum1/2
  [omegak_RSM] -> Gain1/1
  [phik_RSM] -> Sum1/1
  [usk_RSM] -> TP1/1(xk)  "usk_ref"
  Sum1/1 -> TP1/2(phik)
  TP1/1(xs) -> [ussref_RSM]  "uss_ref"
  [ussref_RSM] -> ussref_RSM/1
  [dist_est_log] -> dist_est_log/1

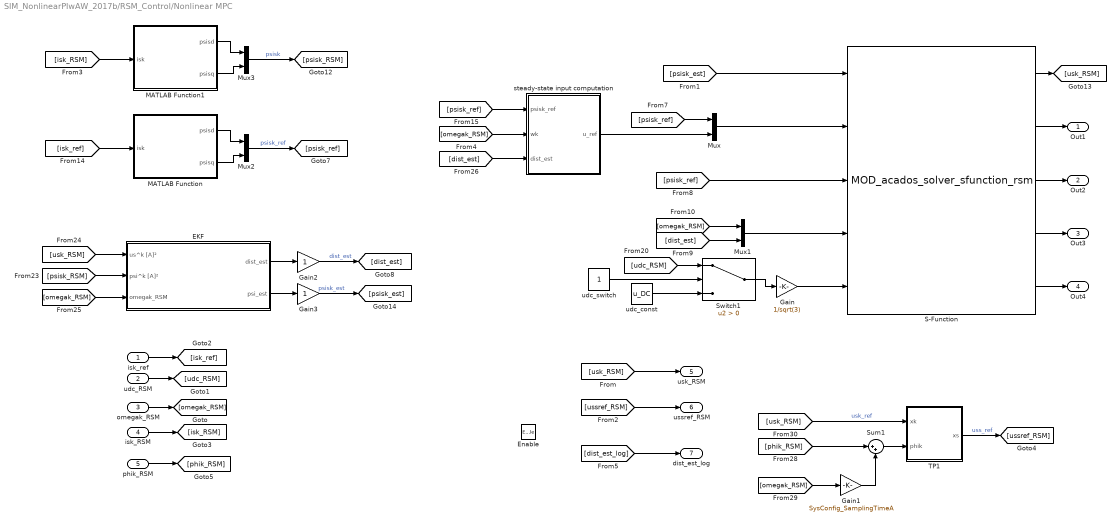
== system SIM_NonlinearPIwAW_2017b/RSM_Control/Nonlinear MPC ==
  isk_ref : Inport
  udc_RSM : Inport  Port=2
  omegak_RSM : Inport  Port=3
  isk_RSM : Inport  Port=4
  phik_RSM : Inport  Port=5
  Enable : EnablePort
  "EKF " : Subsystem
  Gain : Gain  Gain=1/sqrt(3)
  Gain1 : Gain  Gain=SysConfig_SamplingTimeA
  Gain2 : Gain
  Gain3 : Gain
  MATLAB Function : MATLAB Function  TreatAsAtomicUnit=on
  MATLAB Function1 : MATLAB Function  TreatAsAtomicUnit=on
  Mux{,1..3} (4 alike) : Mux  Inputs=2
  S-Function : S-Function  FunctionName=MOD_acados_solver_sfunction_rsm  SFunctionDeploymentMode=off  EnableBusSupport=off
  Sum1 : Sum  Inputs=|++
  Switch1 : Switch  Criteria=u2 > Threshold
  TP1 : MATLAB Function  TreatAsAtomicUnit=on
  steady-state input computation : Subsystem
  udc_const : Constant  Value=u_DC
  udc_switch : Constant
  Out1 : Outport
  Out2 : Outport  Port=2
  Out3 : Outport  Port=3
  Out4 : Outport  Port=4
  usk_RSM : Outport  Port=5
  ussref_RSM : Outport  Port=6
  dist_est_log : Outport  Port=7
  wires:
  S-Function/3 -> Out2/1
  S-Function/1 -> [usk_RSM]
  [psisk_ref] -> steady-state input computation/1(psisk_ref)
  [dist_est] -> steady-state input computation/3(dist_est)
  Gain2/1 -> [dist_est]  "dist_est"
  S-Function/2 -> Out1/1
  [udc_RSM] -> Switch1/1
  [isk_ref] -> MATLAB Function/1(isk)
  [psisk_RSM] -> "EKF "/2(psi^k [A]²)
  [psisk_est] -> S-Function/1
  Mux/1 -> S-Function/2
  Gain/1 -> S-Function/5
  Switch1/1 -> Gain/1
  [dist_est] -> Mux1/2
  [isk_RSM] -> MATLAB Function1/1(isk)
  MATLAB Function1/1(psisd) -> Mux3/1
  [psisk_ref] -> Mux/1
  MATLAB Function1/2(psisq) -> Mux3/2
  S-Function/5 -> Out4/1
  [omegak_RSM] -> "EKF "/3(omegak_RSM)
  [omegak_RSM] -> Mux1/1
  Mux3/1 -> [psisk_RSM]  "psisk"
  udc_switch/1 -> Switch1/2
  MATLAB Function/1(psisd) -> Mux2/1
  [usk_RSM] -> "EKF "/1(us^k [A]²)
  S-Function/4 -> Out3/1
  udc_const/1 -> Switch1/3
  steady-state input computation/1(u_ref) -> Mux/2
  Mux1/1 -> S-Function/4
  Gain3/1 -> [psisk_est]  "psisk_est"
  Mux2/1 -> [psisk_ref]  "psisk_ref"
  "EKF "/1(dist_est) -> Gain2/1
  "EKF "/2(psi_est) -> Gain3/1
  [omegak_RSM] -> steady-state input computation/2(wk)
  MATLAB Function/2(psisq) -> Mux2/2
  [psisk_ref] -> S-Function/3
  isk_ref/1 -> [isk_ref]
  isk_RSM/1 -> [isk_RSM]
  omegak_RSM/1 -> [omegak_RSM]
  phik_RSM/1 -> [phik_RSM]
  udc_RSM/1 -> [udc_RSM]
  [usk_RSM] -> usk_RSM/1
  Gain1/1 -> Sum1/2
  [omegak_RSM] -> Gain1/1
  [phik_RSM] -> Sum1/1
  [usk_RSM] -> TP1/1(xk)  "usk_ref"
  Sum1/1 -> TP1/2(phik)
  TP1/1(xs) -> [ussref_RSM]  "uss_ref"
  [ussref_RSM] -> ussref_RSM/1
  [dist_est_log] -> dist_est_log/1

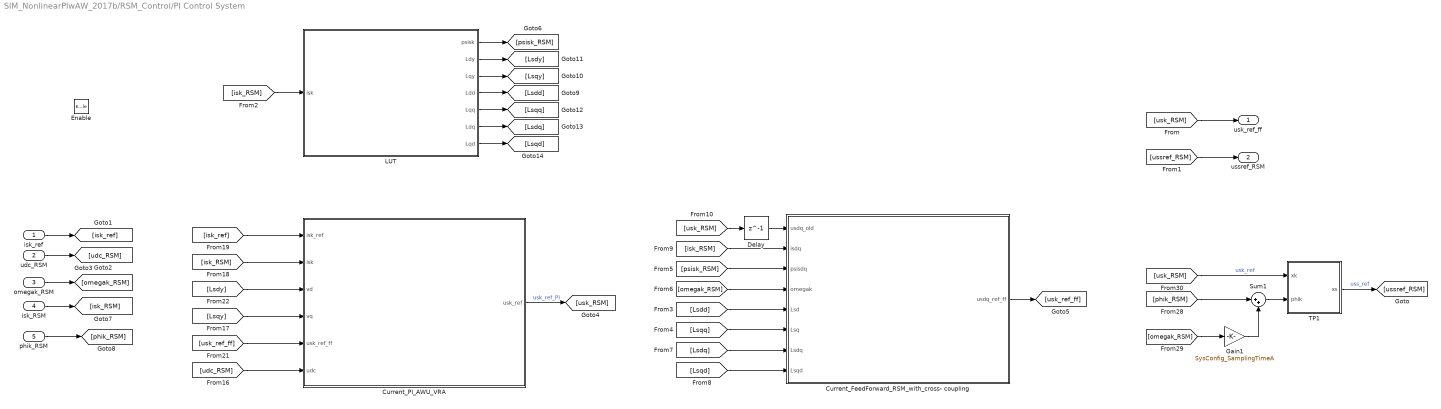
== system SIM_NonlinearPIwAW_2017b/RSM_Control/PI Control System ==
  isk_ref : Inport
  udc_RSM : Inport  Port=2
  omegak_RSM : Inport  Port=3
  isk_RSM : Inport  Port=4
  phik_RSM : Inport  Port=5
  Enable : EnablePort
  Current_FeedForward_RSM_with_cross- coupling : MATLAB Function  TreatAsAtomicUnit=on  mask{RS=rsm_za.Rs}
      mask prompts: RS "Stator resistance (in Ohm)"
  Current_PI_AWU_VRA : Subsystem  mask{VRD=rsm_za.VRis*0.5, TND=rsm_za.Tnis, VRQ=rsm_za.VRis*0.5, TNQ=rsm_za.Tnis}
      mask prompts: VRD "d-Current gain (constant part)"; TND "d-Current time constant (constant part)"; VRQ "q-Current gain (constant part)"; TNQ "q-Current time constant (constant part)"
      mask DialogControl DescGroupVar Prompt: Description
      mask DialogControl DescTextVar Prompt: Current control system with anti windup and online parameter adjustment.
  Delay : Delay  DelayLength=1
  Gain1 : Gain  Gain=SysConfig_SamplingTimeA
  LUT : Subsystem
  Sum1 : Sum  Inputs=|++
  TP1 : MATLAB Function  TreatAsAtomicUnit=on
  usk_ref_ff : Outport
  ussref_RSM : Outport  Port=2
  wires:
  Current_PI_AWU_VRA/1(usk_ref) -> [usk_RSM]  "usk_ref_PI"
  LUT/2(Ldy) -> [Lsdy]
  Gain1/1 -> Sum1/2
  [isk_RSM] -> LUT/1(isk)
  [omegak_RSM] -> Current_FeedForward_RSM_with_cross- coupling/4(omegak)
  [omegak_RSM] -> Gain1/1
  [usk_ref_ff] -> Current_PI_AWU_VRA/5(usk_ref_ff)
  TP1/1(xs) -> [ussref_RSM]  "uss_ref"
  [udc_RSM] -> Current_PI_AWU_VRA/6(udc)
  [Lsqy] -> Current_PI_AWU_VRA/4(vq)
  Sum1/1 -> TP1/2(phik)
  [usk_RSM] -> TP1/1(xk)  "usk_ref"
  [isk_RSM] -> Current_PI_AWU_VRA/2(isk)
  LUT/1(psisk) -> [psisk_RSM]
  [isk_ref] -> Current_PI_AWU_VRA/1(isk_ref)
  LUT/3(Lqy) -> [Lsqy]
  [Lsdy] -> Current_PI_AWU_VRA/3(vd)
  [psisk_RSM] -> Current_FeedForward_RSM_with_cross- coupling/3(psisdq)
  [phik_RSM] -> Sum1/1
  isk_ref/1 -> [isk_ref]
  udc_RSM/1 -> [udc_RSM]
  omegak_RSM/1 -> [omegak_RSM]
  isk_RSM/1 -> [isk_RSM]
  phik_RSM/1 -> [phik_RSM]
  [usk_RSM] -> usk_ref_ff/1
  [ussref_RSM] -> ussref_RSM/1
  Current_FeedForward_RSM_with_cross- coupling/1(usdq_ref_ff) -> [usk_ref_ff]
  LUT/5(Lqq) -> [Lsqq]
  LUT/4(Ldd) -> [Lsdd]
  LUT/6(Ldq) -> [Lsdq]
  LUT/7(Lqd) -> [Lsqd]
  [Lsdd] -> Current_FeedForward_RSM_with_cross- coupling/5(Lsd)
  [Lsqq] -> Current_FeedForward_RSM_with_cross- coupling/6(Lsq)
  [Lsdq] -> Current_FeedForward_RSM_with_cross- coupling/7(Lsdq)
  [Lsqd] -> Current_FeedForward_RSM_with_cross- coupling/8(Lsqd)
  [isk_RSM] -> Current_FeedForward_RSM_with_cross- coupling/2(isdq)
  Delay/1 -> Current_FeedForward_RSM_with_cross- coupling/1(usdq_old)
  [usk_RSM] -> Delay/1

== system SIM_NonlinearPIwAW_2017b/RSM_Control/current trajectory generator ==
  REF_GEN : MATLAB Function  TreatAsAtomicUnit=on
  duration : Constant  Value=0.1
  id_vec : Constant  Value=-0.3*[-10 -15 -20 -25 -30 -35 -37.5 -35 -40 -35 -30 -25]
  iq_vec : Constant  Value=[-10 -15 -20 -25 -30 -35 -37.5 -35 -37.5 -35 -30 -25]
  isk_ref_out : Outport
  wires:
  id_vec/1 -> REF_GEN/1(id_vec)
  REF_GEN/1(isk_ref) -> isk_ref_out/1
  iq_vec/1 -> REF_GEN/2(iq_vec)
  duration/1 -> REF_GEN/3(duration)

== system SIM_NonlinearPIwAW_2017b/RSM_Control/current_trajectory ==
  ENABLE : Inport
  Product : Product
  REF_GEN : MATLAB Function  TreatAsAtomicUnit=on
  duration : Constant  Value=.25
  mmax : Constant  Value=58
  xvecp : Constant  Value=[0 .25 0 -.25 0 .5 0 -.5 0 .75 0 -.75 0 1 0 -1 0]
  xvecp1 : Constant  Value=[0 0.5 0.25 1 0 -1 -0.25 -0.5 0]
  xvecp2 : Constant  Commented=on  Value=[0 0.5 0.25 1 0 -1 -0.25 -0.5 0]
  mmref : Outport
  flag : Outport  Port=2
  wires:
  ENABLE/1 -> REF_GEN/1(ENABLE_FLAG)
  REF_GEN/2(active_flag) -> flag/1
  REF_GEN/1(mmref) -> mmref/1
  xvecp1/1 -> Product/1
  Product/1 -> REF_GEN/2(xvec)
  mmax/1 -> Product/2
  duration/1 -> REF_GEN/3(duration)

== system SIM_NonlinearPIwAW_2017b/PMSM_Control/CurrentPIAWU/d_Current_PI_AWU_VRA ==
  e : Inport
  int_sw : Inport  Port=2
  1/Tn : Gain  Gain=1/TN
  Constant : Constant  Value=0
  Discrete-Time Integrator : DiscreteIntegrator  SampleTime=-1  ICPrevOutput=DiscIntNeverNeededParam  ICPrevScaledInput=DiscIntNeverNeededParam
  Sum : Sum  Inputs=|++
  Switch : Switch  Criteria=u2 > Threshold
  VR : Gain  Gain=VR
  xpi_ref : Outport
  wires:
  VR/1 -> Sum/1, 1/Tn/1
  Discrete-Time Integrator/1 -> Sum/2
  Constant/1 -> Switch/3
  Sum/1 -> xpi_ref/1
  int_sw/1 -> Switch/2
  Switch/1 -> Discrete-Time Integrator/1
  1/Tn/1 -> Switch/1
  e/1 -> VR/1

== system SIM_NonlinearPIwAW_2017b/PMSM_Control/CurrentPIAWU/q_Current_PI_AWU_VRA ==
  e : Inport
  int_sw : Inport  Port=2
  1/Tn : Gain  Gain=1/TN
  Constant : Constant  Value=0
  Discrete-Time Integrator : DiscreteIntegrator  SampleTime=-1  ICPrevOutput=DiscIntNeverNeededParam  ICPrevScaledInput=DiscIntNeverNeededParam
  Sum : Sum  Inputs=|++
  Switch : Switch  Criteria=u2 > Threshold
  VR : Gain  Gain=VR
  xpi_ref : Outport
  wires:
  e/1 -> VR/1
  1/Tn/1 -> Switch/1
  Switch/1 -> Discrete-Time Integrator/1
  int_sw/1 -> Switch/2
  Sum/1 -> xpi_ref/1
  Constant/1 -> Switch/3
  Discrete-Time Integrator/1 -> Sum/2
  VR/1 -> Sum/1, 1/Tn/1

== system SIM_NonlinearPIwAW_2017b/RSM_Control/Christoph's controler/Current Controller (d) ==
  e_i : Inport
  L_tilde : Inport  Port=2
  AWU : Inport  Port=3
  Constant : Constant  Value=0
  Discrete-Time Integrator : DiscreteIntegrator  SampleTime=-1  ICPrevOutput=DiscIntNeverNeededParam  ICPrevScaledInput=DiscIntNeverNeededParam
  Product4 : Product
  Proportional gain : Gain  Gain=P_GAIN
  Sum : Sum
  Switch : Switch  Criteria=u2 > Threshold
  integral gain : Gain  Gain=I_GAIN
  u_pi : Outport
  u_p : Outport  Port=2
  u_i : Outport  Port=3
  wires:
  Constant/1 -> Switch/3
  e_i/1 -> integral gain/1, Proportional gain/1
  Sum/1 -> u_pi/1
  L_tilde/1 -> Product4/1
  Proportional gain/1 -> Product4/2
  Product4/1 -> u_p/1, Sum/1  "u_P"
  integral gain/1 -> Switch/1
  AWU/1 -> Switch/2
  Switch/1 -> Discrete-Time Integrator/1
  Discrete-Time Integrator/1 -> u_i/1, Sum/2

== system SIM_NonlinearPIwAW_2017b/RSM_Control/Christoph's controler/Current Controller (q) ==
  e_i : Inport
  L_tilde : Inport  Port=2
  AWU : Inport  Port=3
  Constant : Constant  Value=0
  Discrete-Time Integrator : DiscreteIntegrator  SampleTime=-1  ICPrevOutput=DiscIntNeverNeededParam  ICPrevScaledInput=DiscIntNeverNeededParam
  Product4 : Product
  Proportional gain : Gain  Gain=P_GAIN
  Sum : Sum
  Switch : Switch  Criteria=u2 > Threshold
  integral gain : Gain  Gain=I_GAIN
  u_pi : Outport
  u_p : Outport  Port=2
  u_i : Outport  Port=3
  wires:
  Discrete-Time Integrator/1 -> Sum/2, u_i/1
  Switch/1 -> Discrete-Time Integrator/1
  AWU/1 -> Switch/2
  integral gain/1 -> Switch/1
  Product4/1 -> Sum/1, u_p/1  "u_P"
  Proportional gain/1 -> Product4/2
  L_tilde/1 -> Product4/1
  Sum/1 -> u_pi/1
  e_i/1 -> Proportional gain/1, integral gain/1
  Constant/1 -> Switch/3

== system SIM_NonlinearPIwAW_2017b/RSM_Control/Christoph's controler/Euclidean norm1 ==
  x [..] : Inport
  Dot Product : DotProduct  InputSameDT=on  OutDataTypeStr=Inherit: Inherit via internal rule
  Sqrt : Sqrt  SaturateOnIntegerOverflow=on
  ||x|| [..] : Outport
  wires:
  x [..]/1 -> Dot Product/1, Dot Product/2
  Dot Product/1 -> Sqrt/1
  Sqrt/1 -> ||x|| [..]/1  "||e(t)|| [..]"

== system SIM_NonlinearPIwAW_2017b/RSM_Control/Christoph's controler/Euclidean norm2 ==
  x [..] : Inport
  Dot Product : DotProduct  InputSameDT=on  OutDataTypeStr=Inherit: Inherit via internal rule
  Sqrt : Sqrt  SaturateOnIntegerOverflow=on
  ||x|| [..] : Outport
  wires:
  Sqrt/1 -> ||x|| [..]/1  "||e(t)|| [..]"
  Dot Product/1 -> Sqrt/1
  x [..]/1 -> Dot Product/2, Dot Product/1

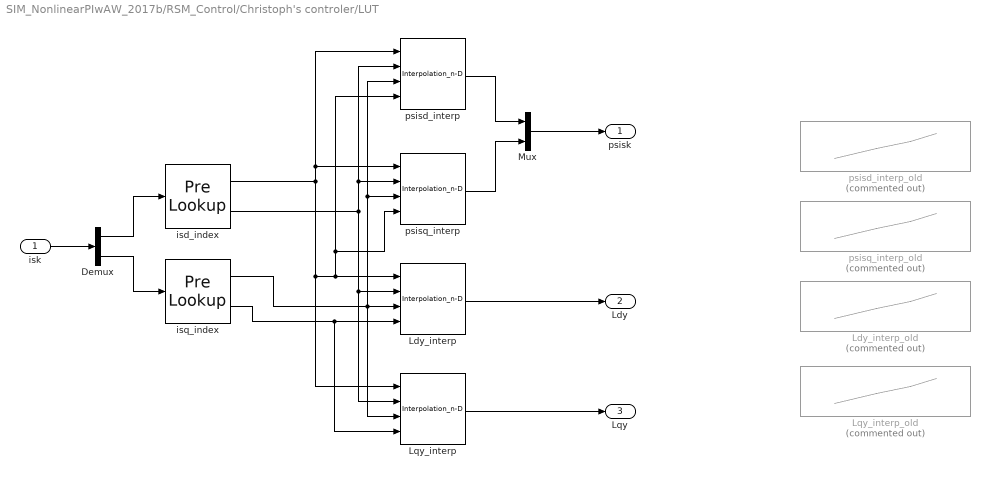
== system SIM_NonlinearPIwAW_2017b/RSM_Control/Christoph's controler/LUT ==
  isk : Inport
  Demux : Demux  Outputs=2
  Ldy_interp : Interpolation_n-D  Table=rsm_za.Ls.dy'  ExtrapMethod=Clip  InternalRulePriority=Speed
  Ldy_interp_old : Lookup_n-D  Commented=on  BreakpointsForDimension1=rsm_za.Is.d(1,:)  BreakpointsForDimension2=rsm_za.Is.q(:,1)  UseOneInputPortForAllInputData=on  Table=rsm_za.Ls.dy'  InternalRulePriority=Speed  RndMeth=Simplest  InputSameDT=on
  Lqy_interp : Interpolation_n-D  Table=rsm_za.Ls.qy'  ExtrapMethod=Clip  InternalRulePriority=Speed
  Lqy_interp_old : Lookup_n-D  Commented=on  BreakpointsForDimension1=rsm_za.Is.d(1,:)  BreakpointsForDimension2=rsm_za.Is.q(:,1)  UseOneInputPortForAllInputData=on  Table=rsm_za.Ls.qy'  InternalRulePriority=Speed  RndMeth=Simplest  InputSameDT=on
  Mux : Mux  Inputs=2
  isd_index : PreLookup  BreakpointsData=rsm_za.Is.d(1,:)  BeginIndexSearchUsingPreviousIndexResult=on  ExtrapMethod=Linear
  isq_index : PreLookup  BreakpointsData=rsm_za.Is.q(:,1)  BeginIndexSearchUsingPreviousIndexResult=on  ExtrapMethod=Linear
  psisd_interp : Interpolation_n-D  Table=rsm_za.Psis.d'  ExtrapMethod=Clip  InternalRulePriority=Speed
  psisd_interp_old : Lookup_n-D  Commented=on  BreakpointsForDimension1=rsm_za.Is.d(1,:)  BreakpointsForDimension2=rsm_za.Is.q(:,1)  UseOneInputPortForAllInputData=on  Table=rsm_za.Psis.d'  InternalRulePriority=Speed  RndMeth=Simplest  InputSameDT=on
  psisq_interp : Interpolation_n-D  Table=rsm_za.Psis.q'  ExtrapMethod=Clip  InternalRulePriority=Speed
  psisq_interp_old : Lookup_n-D  Commented=on  BreakpointsForDimension1=rsm_za.Is.d(1,:)  BreakpointsForDimension2=rsm_za.Is.q(:,1)  UseOneInputPortForAllInputData=on  Table=rsm_za.Psis.q'  InternalRulePriority=Speed  RndMeth=Simplest  InputSameDT=on
  psisk : Outport
  Ldy : Outport  Port=2
  Lqy : Outport  Port=3
  wires:
  psisd_interp/1 -> Mux/1
  psisq_interp/1 -> Mux/2
  Mux/1 -> psisk/1
  Ldy_interp/1 -> Ldy/1
  Lqy_interp/1 -> Lqy/1
  isk/1 -> Demux/1
  Demux/1 -> isd_index/1
  Demux/2 -> isq_index/1
  isd_index/1 -> Lqy_interp/1, psisd_interp/4, psisq_interp/4, Ldy_interp/1, psisq_interp/1, psisd_interp/1
  isd_index/2 -> Lqy_interp/2, Ldy_interp/2, psisd_interp/2, psisq_interp/2
  isq_index/1 -> Lqy_interp/3, psisd_interp/3, psisq_interp/3, Ldy_interp/3
  isq_index/2 -> Lqy_interp/4, Ldy_interp/4

== system SIM_NonlinearPIwAW_2017b/RSM_Control/Christoph's controler/Park transformation x^k -> x^s ==
  x^k : Inport
  phi_k [rad] : Inport  Port=2
  Demux : Demux  Outputs=2
  Mux : Mux  Inputs=2
  Product{,1..3} (4 alike) : Product
  Sum : Sum  Inputs=|+-
  Sum1 : Sum  Inputs=|++
  Trigonometric Function : Trigonometry
  Trigonometric Function1 : Trigonometry  Operator=cos
  x^s : Outport
  wires:
  Mux/1 -> x^s/1
  x^k/1 -> Demux/1
  Sum1/1 -> Mux/2  "x^beta"
  Product3/1 -> Sum1/2  "x^q*cos(phi_k)"
  Product2/1 -> Sum1/1  "x^d*sin(phi_k)"
  Product1/1 -> Sum/2  "x^q*sin(phi_k)"
  Product/1 -> Sum/1  "x^d*cos(phi_k)"
  Trigonometric Function/1 -> Product1/2, Product2/2  "sin(phi_k)"
  Demux/2 -> Product1/1, Product3/1  "x^q"
  Trigonometric Function1/1 -> Product/2, Product3/2  "cos(phi_k)"
  Demux/1 -> Product2/1, Product/1  "x^d"
  phi_k [rad]/1 -> Trigonometric Function1/1, Trigonometric Function/1
  Sum/1 -> Mux/1  "x^alpha"

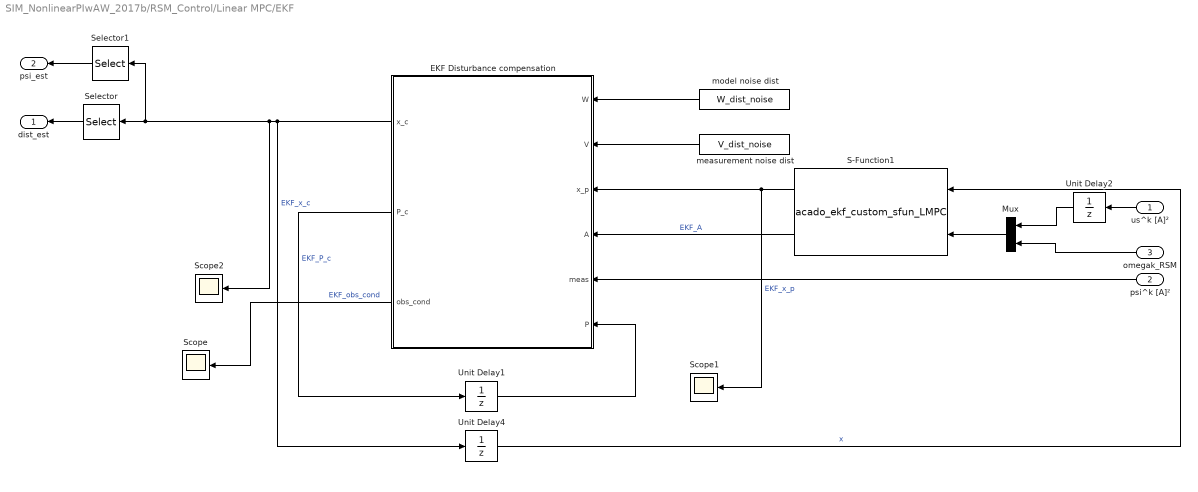
== system SIM_NonlinearPIwAW_2017b/RSM_Control/Linear MPC/EKF  ==
  us^k [A]² : Inport
  psi^k [A]² : Inport  Port=2
  omegak_RSM : Inport  Port=3
  EKF Disturbance compensation : MATLAB Function  TreatAsAtomicUnit=on
  Mux : Mux  Inputs=2
  S-Function1 : S-Function  FunctionName=acado_ekf_custom_sfun_LMPC  Parameters=[0 0 0 0]  SFunctionDeploymentMode=off  EnableBusSupport=off
  Scope : Scope
  Scope1 : Scope
  Scope2 : Scope
  Selector : Selector  InputPortWidth=4  IndexOptions=Index vector (dialog)  Indices=[3 4]  OutputSizes=1
  Selector1 : Selector  InputPortWidth=4  IndexOptions=Index vector (dialog)  Indices=[1 2]  OutputSizes=1
  Unit Delay1 : UnitDelay  InitialCondition=P_init_dist  SampleTime=-1
  Unit Delay2 : UnitDelay  InitialCondition=[0,0]  SampleTime=-1
  Unit Delay4 : UnitDelay  InitialCondition=x_e_init_dist  SampleTime=-1
  measurement noise dist : Constant  Value=V_dist_noise
  model noise dist : Constant  Value=W_dist_noise
  dist_est : Outport
  psi_est : Outport  Port=2
  wires:
  EKF Disturbance compensation/2(P_c) -> Unit Delay1/1  "EKF_P_c"
  measurement noise dist/1 -> EKF Disturbance compensation/2(V)
  EKF Disturbance compensation/3(obs_cond) -> Scope/1  "EKF_obs_cond"
  model noise dist/1 -> EKF Disturbance compensation/1(W)
  Unit Delay4/1 -> S-Function1/1  "x"
  EKF Disturbance compensation/1(x_c) -> Selector1/1, Selector/1, Scope2/1, Unit Delay4/1  "EKF_x_c"
  Unit Delay1/1 -> EKF Disturbance compensation/6(P)
  S-Function1/2 -> EKF Disturbance compensation/4(A)  "EKF_A"
  S-Function1/1 -> Scope1/1, EKF Disturbance compensation/3(x_p)  "EKF_x_p"
  psi^k [A]²/1 -> EKF Disturbance compensation/5(meas)
  Selector/1 -> dist_est/1
  us^k [A]²/1 -> Unit Delay2/1
  omegak_RSM/1 -> Mux/2
  Mux/1 -> S-Function1/2
  Selector1/1 -> psi_est/1
  Unit Delay2/1 -> Mux/1
